simulink subsystem "Day2_Scenario_1"  (R2024a)
settings: Solver=VariableStepAuto  StartTime=0.0  StopTime=10.0  RelTol=1e-3
libraries: CarMaker4SL x2
settings Model: Creator=junhyung.cha  LastModifiedBy=User

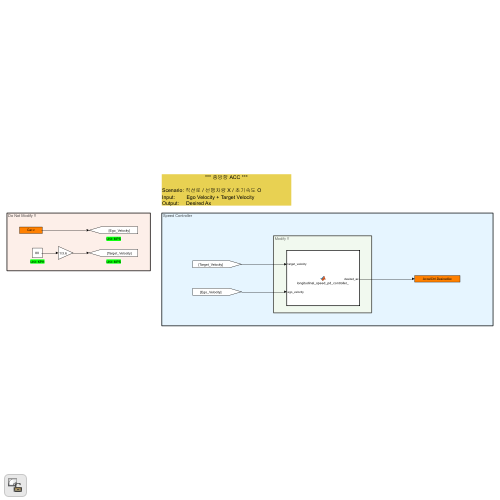
[thumbnail: Simulink's stored preview of the top-level diagram]
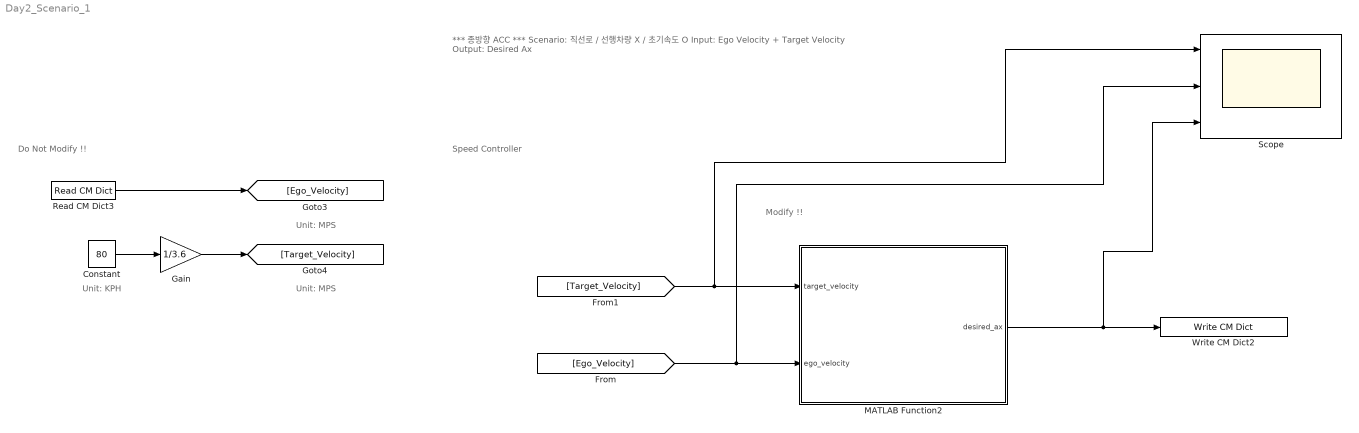
== system Day2_Scenario_1 ==
  note: Unit: KPH
  note: *** 종방향 ACC ***
      |
      | Scenario: 직선로 / 선행차량 X / 초기속도 O
      | Input: Ego Velocity + Target Velocity
      | Output: Desired Ax
  note: Do Not Modify !!
  note: Modify !!
  note: Speed Controller
  note: Unit: MPS
  note: Unit: MPS
  Constant : Constant  Value=80
  Gain : Gain  Gain=1/3.6
  MATLAB Function2 : MATLAB Function  TreatAsAtomicUnit=on
  Read CM Dict3 : CarMaker4SL/Read CM Dict  xname=Car.v  xsync=off  xstime=Inherited
  Scope : Scope  NumInputPorts=3
  Write CM Dict2 : CarMaker4SL/Write CM Dict  xname=AccelCtrl.DesiredAx  xsync=off
  wires:
  MATLAB Function2/1(desired_ax) -> Write CM Dict2/1, Scope/3
  [Target_Velocity] -> MATLAB Function2/1(target_velocity), Scope/1
  Constant/1 -> Gain/1
  [Ego_Velocity] -> MATLAB Function2/2(ego_velocity), Scope/2
  Read CM Dict3/1 -> [Ego_Velocity]
  Gain/1 -> [Target_Velocity]

== matlab function Day2_Scenario_1/MATLAB Function2 ==
  settings: updateMethod=DISCRETE  sampleTime=0.05
  data: target_velocity input; desired_ax output; ego_velocity input
function desired_ax = longitudinal_speed_pd_controller_(target_velocity, ego_velocity)
% PD 제어기: 속도 오차 → 가속도 출력
% 입력:
%   - target_velocity: 목표 속도 [m/s]
%   - ego_velocity: 현재 속도 [m/s]
% 출력:
%   - desired_ax: 원하는 종방향 가속도 [m/s^2]

% --- 내부 상태 유지용 persistent 변수 ---
persistent prev_error
persistent initialized
dt = 0.001;  % 제어 주기 [초]

% --- 초기화 ---
if isempty(initialized)
    prev_error = 0;
    initialized = true;
end

% --- PD 게인 설정 ---
Kp = 10.0;     % 비례 게인
Kd = 0.1;        % 미분 게인

% --- 오차 계산 ---
error = target_velocity - ego_velocity;
d_error = (error - prev_error) / dt;

% --- PD 제어 계산 ---
desired_ax = Kp * error + Kd * d_error;

% --- Saturation 범위 설정 ---
MAX_AX = 10.0;   % 최대 가속도
MIN_AX = -5.0;  % 최대 감속도 (제동)

% --- Saturation 적용 ---
if desired_ax > MAX_AX
    desired_ax = MAX_AX;
elseif desired_ax < MIN_AX
    desired_ax = MIN_AX;
end

% --- 상태 업데이트 ---
prev_error = error;
end
